simulink model "test"  (R2021a)
settings: Solver=VariableStepAuto  StartTime=0.0  StopTime=10.0  RelTol=1e-3
values from neighbouring files (symbols this model uses):
  k = 6    [exercise3.m]
  kp = 0.615    [exercise3.m]
  T_1 = 5.9    [exercise3.m]
  T_2 = 0.8    [exercise3.m]
  Td = 0.1    [exercise3.m]
  Ti = 3.2    [exercise3.m]
  Tp = 0.01    [exercise3.m]
undefined symbols (not defined in the file or in its folder): magnitude
settings Model: Creator=Paweł  LastModifiedBy=Paweł

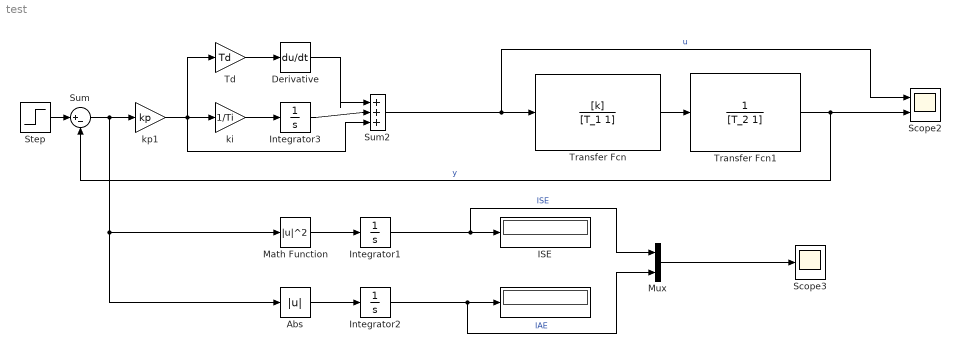
== system test ==
  " " : Display
  Abs : Abs  SaturateOnIntegerOverflow=on
  Derivative : Derivative
  ISE : Display
  Integrator1 : Integrator  InitialCondition=Tp
  Integrator2 : Integrator
  Integrator3 : Integrator
  Math Function : Math  Operator=magnitude^2  SignedPower=on  SaturateOnIntegerOverflow=on
  Mux : Mux  Inputs=2
  Scope2 : Scope  NumInputPorts=2
  Scope3 : Scope
  Step : Step  Time=0  SampleTime=Tp
  Sum : Sum  Inputs=|+-
  Sum2 : Sum  Inputs=|+++  SaturateOnIntegerOverflow=on
  Td : Gain  Gain=Td  SaturateOnIntegerOverflow=on  OutDataTypeStr=Inherit: Same as input  ParamDataTypeStr=Inherit: Same as input
  Transfer Fcn : TransferFcn  Numerator=[k]  Denominator=[T_1 1]
  Transfer Fcn1 : TransferFcn  Denominator=[T_2 1]
  ki : Gain  Gain=1/Ti  SaturateOnIntegerOverflow=on  OutDataTypeStr=Inherit: Same as input  ParamDataTypeStr=Inherit: Same as input
  kp1 : Gain  Gain=kp  SaturateOnIntegerOverflow=on  OutDataTypeStr=Inherit: Same as input  ParamDataTypeStr=Inherit: Same as input
  wires:
  Derivative/1 -> Sum2/1
  kp1/1 -> Td/1, Sum2/3, ki/1
  Sum2/1 -> Transfer Fcn/1, Scope2/1  "u"
  Transfer Fcn1/1 -> Sum/2, Scope2/2  "y"
  Integrator1/1 -> Mux/1, ISE/1  "ISE"
  Td/1 -> Derivative/1
  Integrator3/1 -> Sum2/2
  ki/1 -> Integrator3/1
  Mux/1 -> Scope3/1
  Sum/1 -> kp1/1, Math Function/1, Abs/1
  Transfer Fcn/1 -> Transfer Fcn1/1
  Integrator2/1 -> Mux/2, " "/1  "IAE"
  Abs/1 -> Integrator2/1
  Math Function/1 -> Integrator1/1
  Step/1 -> Sum/1
